simulink model "R2015a_AccBasedControl"  (R2015a)
settings: Solver=ode45  SolverMode=SingleTasking  StartTime=0.0  StopTime=10  RelTol=1e-3
libraries: simulink x2
settings Model: CovMetricSettings=dwe  CovHtmlReporting=off  covSaveCumulativeToWorkspaceVar=off  CovSaveSingleToWorkspaceVar=off  CovExternalEMLEnable=on  Creator=leonardof  LastModifiedBy=Leonardo Felipe
settings DataIOCC: LimitDataPoints=off  SaveFormat=Dataset
settings DebuggingCC: SFUnexpectedBacktrackingDiag=error  SFNoUnconditionalDefaultTransitionDiag=error
settings HardwareCC: ProdBitPerPointer=64  ProdLargestAtomicFloat=Float  ProdIntDivRoundTo=Zero  ProdEndianess=LittleEndian  ProdHWDeviceType=Specified
settings ModelReferenceCC: PropagateSignalLabelsOutOfModel=on
settings GRTTargetCC: TargetLangStandard=C99 (ISO)  GeneratePreprocessorConditionals=Use local settings

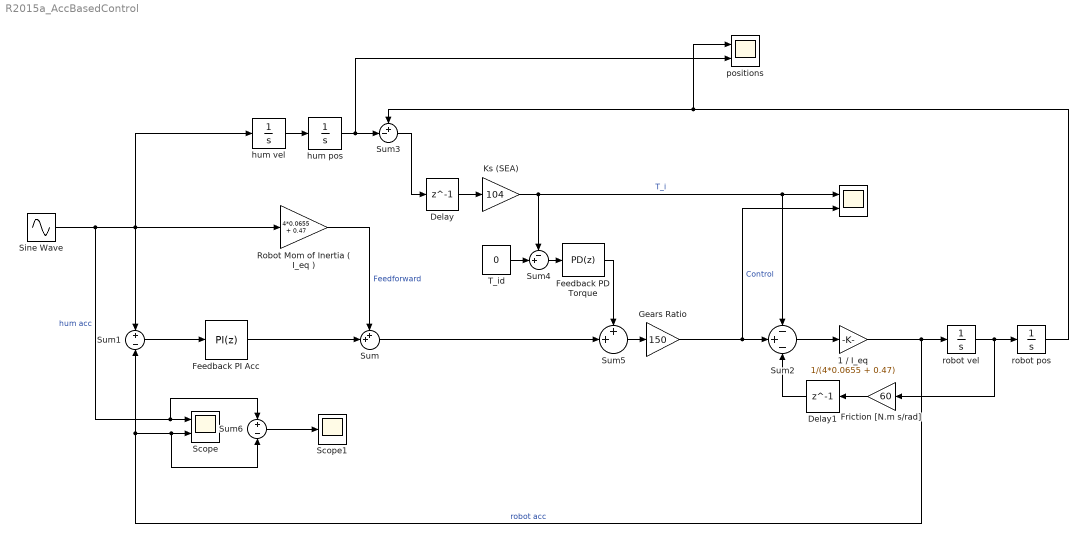
== system R2015a_AccBasedControl ==
  " " : Scope  NumInputPorts=2
      settings: ShowLegends=on  YMin=-400~-1100  YMax=400~1100
  1 / I_eq : Gain  Gain=1/(4*0.0655 + 0.47)
  Delay : Delay  DelayLength=1  InitialCondition=0  SampleTime=0.008333
  Delay1 : Delay  DelayLength=1  InitialCondition=0  SampleTime=0.008333
  Feedback PD Torque : simulink/Continuous/PID Controller  Controller=PD  TimeDomain=Discrete-time  SampleTime=0.008333  IntegratorMethod=Forward Euler  FilterMethod=Forward Euler  Form=Parallel  UseFilter=on  ControllerParametersSource=internal  P=0.004062  I=1  D=0.0076  N=100  InitialConditionSource=internal  InitialConditionForIntegrator=0  InitialConditionForFilter=0  ExternalReset=none  LimitOutput=off  UpperSaturationLimit=inf  LowerSaturationLimit=-inf  LinearizeAsGain=off  AntiWindupMode=none  Kb=1  TrackingMode=off  Kt=1  PParamMin=[]  PParamMax=[]  IParamMin=[]  IParamMax=[]  DParamMin=[]  DParamMax=[]  NParamMin=[]  NParamMax=[]  KbParamMin=[]  KbParamMax=[]  KtParamMin=[]  KtParamMax=[]  POutMin=[]  POutMax=[]  IOutMin=[]  IOutMax=[]  DOutMin=[]  DOutMax=[]  NOutMin=[]  NOutMax=[]  KbOutMin=[]  KbOutMax=[]  KtOutMin=[]  KtOutMax=[]  IntegratorOutMin=[]  IntegratorOutMax=[]  FilterOutMin=[]  FilterOutMax=[]  SumOutMin=[]  SumOutMax=[]  SumI1OutMin=[]  SumI1OutMax=[]  SumI2OutMin=[]  SumI2OutMax=[]  SumI3OutMin=[]  SumI3OutMax=[]  SumDOutMin=[]  SumDOutMax=[]  SaturationOutMin=[]  SaturationOutMax=[]  IntegratorContinuousStateAttributes=''  IntegratorStateMustResolveToSignalObject=off  IntegratorRTWStateStorageClass=Auto  FilterContinuousStateAttributes='torque'  FilterStateMustResolveToSignalObject=off  FilterRTWStateStorageClass=Auto  DifferentiatorICPrevScaledInput=0  DifferentiatorOutMin=[]  DifferentiatorOutMax=[]
  Feedback PI Acc : simulink/Continuous/PID Controller  Controller=PI  TimeDomain=Discrete-time  SampleTime=0.008333  IntegratorMethod=Forward Euler  FilterMethod=Forward Euler  Form=Parallel  UseFilter=on  ControllerParametersSource=internal  P=36.82334820843  I=0.0195714639058397  D=0  N=100  InitialConditionSource=internal  InitialConditionForIntegrator=0  InitialConditionForFilter=0  ExternalReset=none  LimitOutput=off  UpperSaturationLimit=inf  LowerSaturationLimit=-inf  LinearizeAsGain=off  AntiWindupMode=none  Kb=1  TrackingMode=off  Kt=1  PParamMin=[]  PParamMax=[]  IParamMin=[]  IParamMax=[]  DParamMin=[]  DParamMax=[]  NParamMin=[]  NParamMax=[]  KbParamMin=[]  KbParamMax=[]  KtParamMin=[]  KtParamMax=[]  POutMin=[]  POutMax=[]  IOutMin=[]  IOutMax=[]  DOutMin=[]  DOutMax=[]  NOutMin=[]  NOutMax=[]  KbOutMin=[]  KbOutMax=[]  KtOutMin=[]  KtOutMax=[]  IntegratorOutMin=[]  IntegratorOutMax=[]  FilterOutMin=[]  FilterOutMax=[]  SumOutMin=[]  SumOutMax=[]  SumI1OutMin=[]  SumI1OutMax=[]  SumI2OutMin=[]  SumI2OutMax=[]  SumI3OutMin=[]  SumI3OutMax=[]  SumDOutMin=[]  SumDOutMax=[]  SaturationOutMin=[]  SaturationOutMax=[]  IntegratorContinuousStateAttributes=''  IntegratorStateMustResolveToSignalObject=off  IntegratorRTWStateStorageClass=Auto  FilterContinuousStateAttributes=''  FilterStateMustResolveToSignalObject=off  FilterRTWStateStorageClass=Auto  DifferentiatorICPrevScaledInput=0  DifferentiatorOutMin=[]  DifferentiatorOutMax=[]
  Friction [N.m s/rad] : Gain  Gain=60
  Gears Ratio : Gain  Gain=150
  Ks (SEA) : Gain  Gain=104
  "Robot Mom of Inertia ( I_eq ) " : Gain  Gain=4*0.0655 + 0.47
  Scope : Scope  NumInputPorts=2
      settings: TimeRange=10  YMin=-25~-20  YMax=25~20
  Scope1 : Scope
      settings: YMin=-0.3  YMax=0.3  SaveName=ScopeData3
  Sine Wave : Sin  Amplitude=20  Frequency=6.28318  SampleTime=0
  Sum : Sum  Inputs=++|
  Sum1 : Sum  Inputs=+|-
  Sum2 : Sum  Inputs=-+-
  Sum3 : Sum  Inputs=+-|
  Sum4 : Sum  Inputs=-+|
  Sum5 : Sum  Inputs=++|
  Sum6 : Sum  Inputs=+|-
  T_id : Constant  Value=0
  hum pos : Integrator  LimitOutput=on  UpperSaturationLimit=3.14159  LowerSaturationLimit=-3.14159  ContinuousStateAttributes='position'
  hum vel : Integrator  InitialCondition=-20/6.28318  LimitOutput=on  UpperSaturationLimit=21  LowerSaturationLimit=-21  ContinuousStateAttributes='velocity'
  positions : Scope  NumInputPorts=2
      settings: ShowLegends=on  YMin=-3.46243~-5  YMax=3.87537~5  SaveName=ScopeData2
  robot pos : Integrator  LimitOutput=on  UpperSaturationLimit=3.14159  LowerSaturationLimit=-3.14159  ContinuousStateAttributes='position'
  robot vel : Integrator  InitialCondition=-20/6.28318  LimitOutput=on  UpperSaturationLimit=21  LowerSaturationLimit=-21  ContinuousStateAttributes='velocity'
  wires:
  Sine Wave/1 -> Sum6/1, Scope/1, hum vel/1, Sum1/1, "Robot Mom of Inertia ( I_eq ) "/1  "hum acc"
  "Robot Mom of Inertia ( I_eq ) "/1 -> Sum/1  "Feedforward"
  Sum2/1 -> 1 / I_eq/1
  hum vel/1 -> hum pos/1
  robot vel/1 -> robot pos/1, Friction [N.m s/rad]/1
  hum pos/1 -> positions/2, Sum3/2
  Ks (SEA)/1 -> Sum4/1, " "/1, Sum2/1  "T_i"
  robot pos/1 -> positions/1, Sum3/1
  Feedback PI Acc/1 -> Sum/2
  Sum1/1 -> Feedback PI Acc/1
  T_id/1 -> Sum4/2
  Sum4/1 -> Feedback PD Torque/1
  Feedback PD Torque/1 -> Sum5/1
  Sum/1 -> Sum5/2
  Sum5/1 -> Gears Ratio/1
  Gears Ratio/1 -> " "/2, Sum2/2  "Control"
  1 / I_eq/1 -> robot vel/1, Sum6/2, Scope/2, Sum1/2  "robot acc"
  Delay/1 -> Ks (SEA)/1
  Sum3/1 -> Delay/1
  Friction [N.m s/rad]/1 -> Delay1/1
  Delay1/1 -> Sum2/3
  Sum6/1 -> Scope1/1
